simulink model "parte5_ej2_GEPs_0228"  (R2019b)
settings: Solver=VariableStepAuto  StartTime=0.0  StopTime=10.0  RelTol=1e-3
values from neighbouring files (symbols this model uses):
  K2 = 0.95567    [parte5_ej2_GEPs_data0228.m]    (also in parte5_eje2_sintonizacionPSS.m = Lads/(Lads+Lfd)*(RT/D*eqo+(XTQ*(xq-xpd)/D+1)*iqo))
  K3 = 0.34284    [parte5_ej2_GEPs_data0228.m]    (also in parte5_eje2_sintonizacionPSS.m = (Lads+Lfd)/Ladu*1/(1+XTQ/D*(xd+xpd)))
  K6 = 0.070874    [parte5_ej2_GEPs_data0228.m]    (also in parte5_eje2_sintonizacionPSS.m = xe*(vqo/Et)/(xe+xpd))
  Ka = 200    [parte5_ej2_GEPs_data0228.m]
  Ke = 1    [parte5_ej2_GEPs_data0228.m]
  T1a = 0    [parte5_ej2_GEPs_data0228.m]
  T2a = 0.1    [parte5_ej2_GEPs_data0228.m]
  T3 = 0.5    [parte5_ej1_PSS_0228.m]    (also in parte5_ej2_GEPs_data0228.m = 2.74272; parte5_eje1_caracteristicasPSS.m = 0.3; parte5_eje2_sintonizacionPSS.m = 0.3)
  Te = 0.01    [parte5_ej2_GEPs_data0228.m]
  Tr = 0.01    [parte5_ej2_GEPs_data0228.m]    (also in parte5_eje2_sintonizacionPSS.m)
settings Model: Creator=cjuar  LastModifiedBy=cjuar

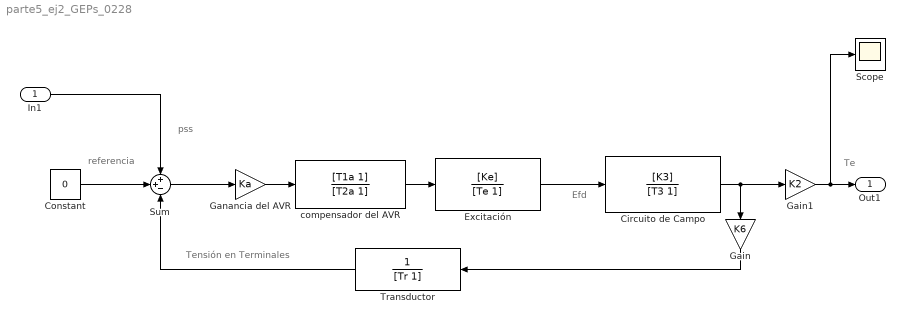
== system parte5_ej2_GEPs_0228 ==
  note: referencia
  note: pss
  note: Te
  note: Efd
  note: Tensión en Terminales
  In1 : Inport
  Circuito de Campo : TransferFcn  Numerator=[K3]  Denominator=[T3 1]
  Constant : Constant  Value=0
  Excitación : TransferFcn  Numerator=[Ke]  Denominator=[Te 1]
  Gain : Gain  Gain=K6
  Gain1 : Gain  Gain=K2
  Ganancia del AVR : Gain  Gain=Ka
  Scope : Scope
  Sum : Sum  Inputs=++-
  Transductor : TransferFcn  Denominator=[Tr 1]
  compensador del AVR : TransferFcn  Numerator=[T1a 1]  Denominator=[T2a 1]
  Out1 : Outport
  wires:
  Excitación/1 -> Circuito de Campo/1
  Ganancia del AVR/1 -> compensador del AVR/1
  compensador del AVR/1 -> Excitación/1
  Circuito de Campo/1 -> Gain1/1, Gain/1
  Gain/1 -> Transductor/1
  Transductor/1 -> Sum/3
  Sum/1 -> Ganancia del AVR/1
  Constant/1 -> Sum/2
  In1/1 -> Sum/1
  Gain1/1 -> Scope/1, Out1/1
